simulink model "ME416_Autonomy_Model"  (R2025b)
settings: Solver=FixedStepAuto  StartTime=0.0  StopTime=20  RelTol=1e-3  EnableMultiTasking=on
PreLoadFcn:
  | driveparam
values from neighbouring files (symbols this model uses):
  alpha_w = 0.7    [driveparam.m]
  beta = Ts / (Ts + tau)    (= 0.166666666667)    [driveparam.m]
  bm = 2e-4    (= 0.0002)    [driveparam.m]
  enable_cmd = 1    [driveparam.m]
  estop_cmd = 0    [driveparam.m]
  Jm = 2e-5    (= 2e-05)    [driveparam.m]
  K_lqr_w = dlqr(Ad_w, Bd_w, Qw, Rw)    [driveparam.m]
  Ke = 0.03    [driveparam.m]
  Kt = 0.03    [driveparam.m]
  L = 0.15    [driveparam.m]
  Lm = 1    [driveparam.m]
  N = 4400    [driveparam.m]
  Nbar_lqr_w = (1 - Ad_w)/Bd_w + K_lqr_w    [driveparam.m]
  r = 0.03    [driveparam.m]
  Rm = 8    [driveparam.m]
  Ts = 0.01    [driveparam.m]
  v_ref_cmd = 0    [driveparam.m]
  Vbatt = 12    [driveparam.m]
  w_ref_cmd = 0.1    [driveparam.m]
undefined symbols (not defined in the file or in its folder): DiscIntNeverNeededParam
libraries: raspberrypiBasiclib x10, raspberrypiCommlib x5, simulink x4, slpidlib x2
settings Model: ExtModeTrigDuration=2  Creator=madak  LastModifiedBy=madak
settings SolverCC: PositivePriorityOrder=on  AutoInsertRateTranBlk=on
settings OptimizationCC: DefaultParameterBehavior=Inlined  EnhancedBackFolding=on  PassReuseOutputArgsAs=Individual arguments  ZeroExternalMemoryAtStartup=off  ZeroInternalMemoryAtStartup=off  MaxStackSize=200000  OptimizeBlockOrder=speed  DifferentSizesBufferReuse=on  OptimizationCustomize=off  EfficientTunableParamExpr=on
settings DebuggingCC: ParameterPrecisionLossMsg=none  ParameterTunabilityLossMsg=error
settings HardwareCC: ProdBitPerLong=64.0  ProdLargestAtomicInteger=LongLong  ProdLargestAtomicFloat=Double  ProdLongLongMode=on  ProdHWDeviceType=ARM Compatible->ARM Cortex-A (64-bit)
settings RTWCC: SystemTargetFile=ert.tlc  HardwareBoard=Raspberry Pi (64bit)  TLCOptions="-aInlineSetEventsForThisBaseRateFcn=TLC_FALSE -aSuppressMultiTaskScheduler=TLC_FALSE  -aRateBasedStepFcn=0"  TemplateMakefile=ert_default_tmf  Toolchain=GNU GCC Embedded Linux  BuildConfiguration=Faster Runs  GPUComputeCapability=3.5  Description=Embedded Coder
settings CodeAppCC: ForceParamTrailComments=on  IgnoreCustomStorageClasses=off  OperatorAnnotations=on  SimulinkDataObjDesc=on  SFDataObjDesc=on  InsertBlockDesc=on
settings ERTTargetCC: ExtModeTransport=2.0  ExtModeStaticAlloc=on  ExtModeMexFile=ext_xcp  ExtModeIntrfLevel=Level2 - Open  RootIOFormat=Structure reference  DynamicArrayContainerType=coder::array  TargetLangStandard=C99 (ISO)  SupportContinuousTime=on  SupportVariableSizeSignals=on

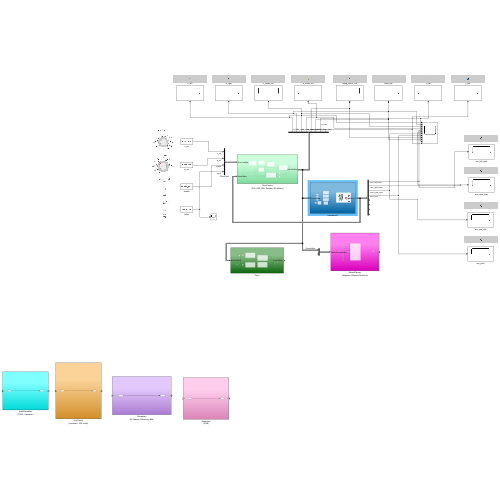
[thumbnail: Simulink's stored preview of the top-level diagram]
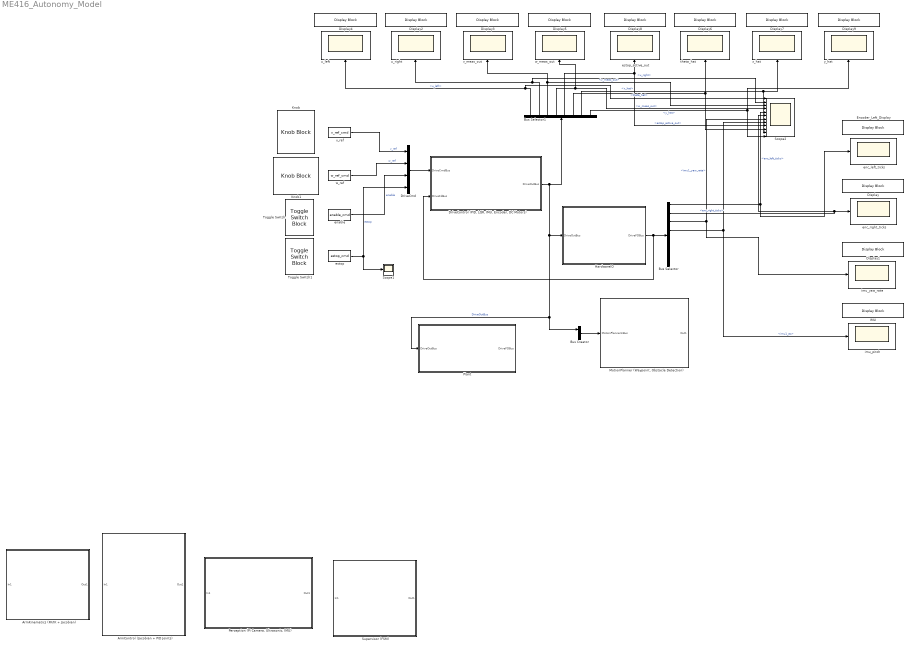
== system ME416_Autonomy_Model ==
  ArmControl (Jacobian + PID Joints) : Subsystem
  ArmKinematics (FK/IK + Jacobian) : Subsystem
  Bus Creator : BusCreator  Inputs=2
  Bus Selector : BusSelector  OutputSignals=enc_left_ticks,enc_right_ticks,imu1_yaw_rate,imu1_az,imu1_ay,imu1_ax,imu1_roll,imu1_pitch
  Bus Selector1 : BusSelector  OutputSignals=u_left,u_right,v_meas_out,w_meas_out,estop_active_out,theta_hat,x_hat,y_hat
  Display{,1..9} (10 alike) : DisplayBlock  LabelPosition=Hide  Transparency=1  GridColor=[0.502, 0.502, 0.502]
  DriveCmd : BusCreator  Inputs=4
  "DriveControl (PID, LQR, IMU, Encoder, DC Motors)" : Subsystem
  Encoder_Left_Display : DisplayBlock  LabelPosition=Hide  Transparency=1  GridColor=[0.502, 0.502, 0.502]
  HardwareIO : Subsystem
  IMU : DisplayBlock  LabelPosition=Hide  Transparency=1  GridColor=[0.502, 0.502, 0.502]
  Knob : KnobBlock  ScaleMin=-0.5  ScaleMax=0.5  TickInterval=0.1
  Knob1 : KnobBlock  ScaleMin=-1  ScaleMax=1
  "MotionPlanner (Waypoint, Obstacle Detection)" : Subsystem
  "Perception (Pi Camera, Ultrasonic, IMU)" : Subsystem
  Plant : Subsystem
  Scope1 : Scope
      settings: ActiveDisplayYMinimum=-1  ActiveDisplayYMaximum=1  DataLoggingVariableName=ScopeData6
  Scope2 : Scope  NumInputPorts=12
      settings: ActiveDisplayYMinimum=-1.25  ActiveDisplayYMaximum=1.25
  Supervisor (FSM) : Subsystem
  Toggle Switch : ToggleSwitchBlock
  Toggle Switch1 : ToggleSwitchBlock
  enable : Constant  Value=enable_cmd
  enc_left_ticks : Scope
      settings: ActiveDisplayYMinimum=-6650.75  ActiveDisplayYMaximum=55596.75
  enc_right_ticks : Scope
      settings: ActiveDisplayYMinimum=-6176.5  ActiveDisplayYMaximum=50648.5  DataLoggingVariableName=ScopeData2
  estop : Constant  Value=estop_cmd  OutDataTypeStr=boolean
  estop_active_out : Scope
      settings: ActiveDisplayYMinimum=-1.25  ActiveDisplayYMaximum=1.25
  imu_pitch : Scope
      settings: ActiveDisplayYMinimum=-1  ActiveDisplayYMaximum=1  DataLoggingVariableName=ScopeData4
  imu_yaw_rate : Scope
      settings: ActiveDisplayYMinimum=-1  ActiveDisplayYMaximum=1  DataLoggingVariableName=ScopeData3
  theta_hat : Scope
      settings: ActiveDisplayYMinimum=-1.25  ActiveDisplayYMaximum=1.25  DataLoggingVariableName=ScopeData2
  u_left : Scope
      settings: ActiveDisplayYMinimum=-1.25  ActiveDisplayYMaximum=1.25
  u_right : Scope
      settings: ActiveDisplayYMinimum=-1.25  ActiveDisplayYMaximum=1.25  DataLoggingVariableName=ScopeData2
  v_meas_out : Scope
      settings: ActiveDisplayYMinimum=-0.06499  ActiveDisplayYMaximum=0.58495  DataLoggingVariableName=ScopeData3
  v_ref : Constant  Value=v_ref_cmd
  w_meas_out : Scope
      settings: ActiveDisplayYMinimum=-29.4564  ActiveDisplayYMaximum=29.55132  DataLoggingVariableName=ScopeData4
  w_ref : Constant  Value=w_ref_cmd
  x_hat : Scope
      settings: ActiveDisplayYMinimum=-6600.125  ActiveDisplayYMaximum=55141.125  DataLoggingVariableName=ScopeData3
  y_hat : Scope
      settings: ActiveDisplayYMinimum=-29.4564  ActiveDisplayYMaximum=29.55132  DataLoggingVariableName=ScopeData4
  wires:
  DriveCmd/1 -> "DriveControl (PID, LQR, IMU, Encoder, DC Motors)"/1(DriveCmdBus)
  "DriveControl (PID, LQR, IMU, Encoder, DC Motors)"/1(DriveOutBus) -> Bus Creator/1, Plant/1(DriveOutBus), HardwareIO/1(DriveOutBus), Bus Selector1/1  "DriveOutBus"
  v_ref/1 -> DriveCmd/1  "v_ref"
  w_ref/1 -> DriveCmd/2  "w_ref"
  enable/1 -> DriveCmd/3  "enable"
  estop/1 -> DriveCmd/4, Scope1/1  "estop"
  Bus Selector/1 -> enc_left_ticks/1, Scope2/5  "<enc_left_ticks>"
  Bus Selector/2 -> Scope2/6, enc_right_ticks/1  "<enc_right_ticks>"
  Bus Selector1/1 -> Scope2/1, u_left/1  "<u_left>"
  Bus Selector1/2 -> Scope2/2, u_right/1  "<u_right>"
  Bus Selector1/3 -> Scope2/3, v_meas_out/1  "<v_meas_out>"
  Bus Selector1/4 -> Scope2/4, w_meas_out/1  "<w_meas_out>"
  Bus Creator/1 -> "MotionPlanner (Waypoint, Obstacle Detection)"/1(MotionPlannerInBus)
  Bus Selector1/5 -> Scope2/9, estop_active_out/1  "<estop_active_out>"
  Bus Selector1/6 -> Scope2/10, theta_hat/1  "<theta_hat>"
  Bus Selector1/7 -> Scope2/11, x_hat/1  "<x_hat>"
  Bus Selector1/8 -> y_hat/1, Scope2/12  "<y_hat>"
  HardwareIO/1("DriveFDBus ") -> "DriveControl (PID, LQR, IMU, Encoder, DC Motors)"/2(DriveFdBus), Bus Selector/1
  Bus Selector/3 -> imu_yaw_rate/1, Scope2/7  "<imu1_yaw_rate>"
  Bus Selector/4 -> imu_pitch/1, Scope2/8  "<imu1_az>"

== system ME416_Autonomy_Model/ArmControl (Jacobian + PID Joints) ==
  In1 : Inport
  Out1 : Outport
  wires:
  In1/1 -> Out1/1

== system ME416_Autonomy_Model/ArmKinematics (FK//IK + Jacobian) ==
  In1 : Inport
  Out1 : Outport
  wires:
  In1/1 -> Out1/1

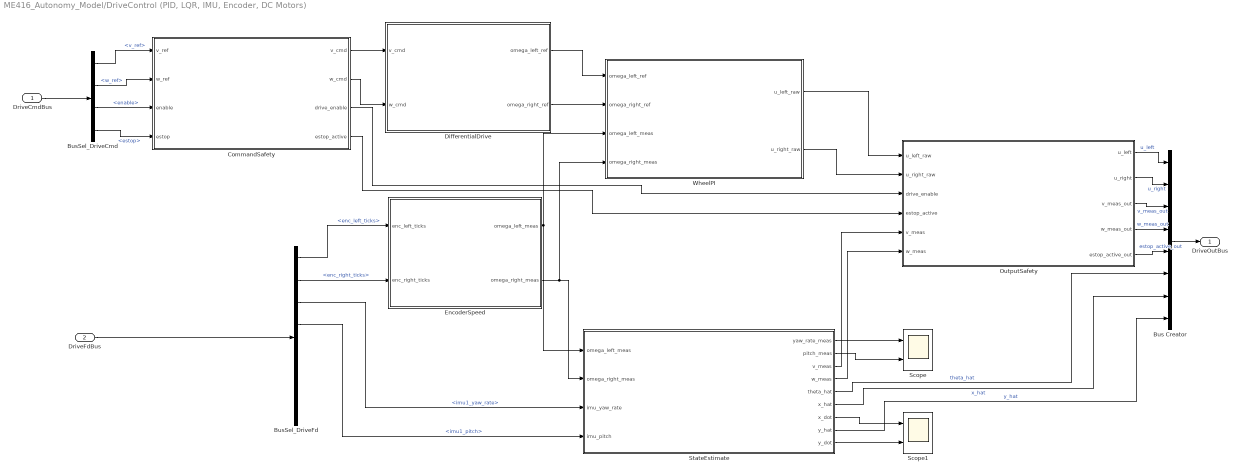
== system ME416_Autonomy_Model/DriveControl (PID, LQR, IMU, Encoder, DC Motors) ==
  DriveCmdBus : Inport
  DriveFdBus : Inport  Port=2
  Bus Creator : BusCreator  Inputs=8
  BusSel_DriveCmd : BusSelector  OutputSignals=v_ref,w_ref,enable,estop
  BusSel_DriveFd : BusSelector  OutputSignals=enc_left_ticks,enc_right_ticks,imu1_yaw_rate,imu1_pitch,imu1_roll,imu1_ax,imu1_ay,imu1_az
  CommandSafety : Subsystem
  DifferentialDrive : Subsystem
  EncoderSpeed : Subsystem
  OutputSafety : Subsystem
  Scope : Scope  NumInputPorts=2
      settings: ActiveDisplayYMinimum=-1  ActiveDisplayYMaximum=1
  Scope1 : Scope  NumInputPorts=2
      settings: ActiveDisplayYMinimum=-1  ActiveDisplayYMaximum=1
  StateEstimate : Subsystem
  WheelPI : Subsystem
  DriveOutBus : Outport
  wires:
  DriveCmdBus/1 -> BusSel_DriveCmd/1
  StateEstimate/4(w_meas) -> OutputSafety/6(w_meas)
  DriveFdBus/1 -> BusSel_DriveFd/1
  StateEstimate/6(x_hat) -> Bus Creator/7  "x_hat"
  BusSel_DriveCmd/1 -> CommandSafety/1(v_ref)  "<v_ref>"
  CommandSafety/2(w_cmd) -> DifferentialDrive/2(w_cmd)
  BusSel_DriveCmd/2 -> CommandSafety/2(w_ref)  "<w_ref>"
  BusSel_DriveCmd/4 -> CommandSafety/4(estop)  "<estop>"
  BusSel_DriveCmd/3 -> CommandSafety/3(enable)  "<enable>"
  CommandSafety/1(v_cmd) -> DifferentialDrive/1(v_cmd)
  CommandSafety/3(drive_enable) -> OutputSafety/3(drive_enable)
  CommandSafety/4(estop_active) -> OutputSafety/4(estop_active)
  StateEstimate/3(v_meas) -> OutputSafety/5(v_meas)
  BusSel_DriveFd/1 -> EncoderSpeed/1(enc_left_ticks)  "<enc_left_ticks>"
  BusSel_DriveFd/2 -> EncoderSpeed/2(enc_right_ticks)  "<enc_right_ticks>"
  BusSel_DriveFd/3 -> StateEstimate/3(imu_yaw_rate)  "<imu1_yaw_rate>"
  BusSel_DriveFd/4 -> StateEstimate/4(imu_pitch)  "<imu1_pitch>"
  DifferentialDrive/1(omega_left_ref) -> WheelPI/1(omega_left_ref)
  DifferentialDrive/2(omega_right_ref) -> WheelPI/2(omega_right_ref)
  EncoderSpeed/1(omega_left_meas) -> StateEstimate/1(omega_left_meas), WheelPI/3(omega_left_meas)
  EncoderSpeed/2(omega_right_meas) -> WheelPI/4(omega_right_meas), StateEstimate/2(omega_right_meas)
  WheelPI/1(u_left_raw) -> OutputSafety/1(u_left_raw)
  WheelPI/2(u_right_raw) -> OutputSafety/2(u_right_raw)
  Bus Creator/1 -> DriveOutBus/1
  StateEstimate/9(y_dot) -> Scope1/2
  StateEstimate/1(yaw_rate_meas) -> Scope/1
  StateEstimate/2(pitch_meas) -> Scope/2
  StateEstimate/5(theta_hat) -> Bus Creator/6  "theta_hat"
  StateEstimate/7(x_dot) -> Scope1/1
  StateEstimate/8(y_hat) -> Bus Creator/8  "y_hat"
  OutputSafety/1(u_left) -> Bus Creator/1  "u_left"
  OutputSafety/2(u_right) -> Bus Creator/2  "u_right"
  OutputSafety/3(v_meas_out) -> Bus Creator/3  "v_meas_out"
  OutputSafety/4(w_meas_out) -> Bus Creator/4  "w_meas_out"
  OutputSafety/5(estop_active_out) -> Bus Creator/5  "estop_active_out"

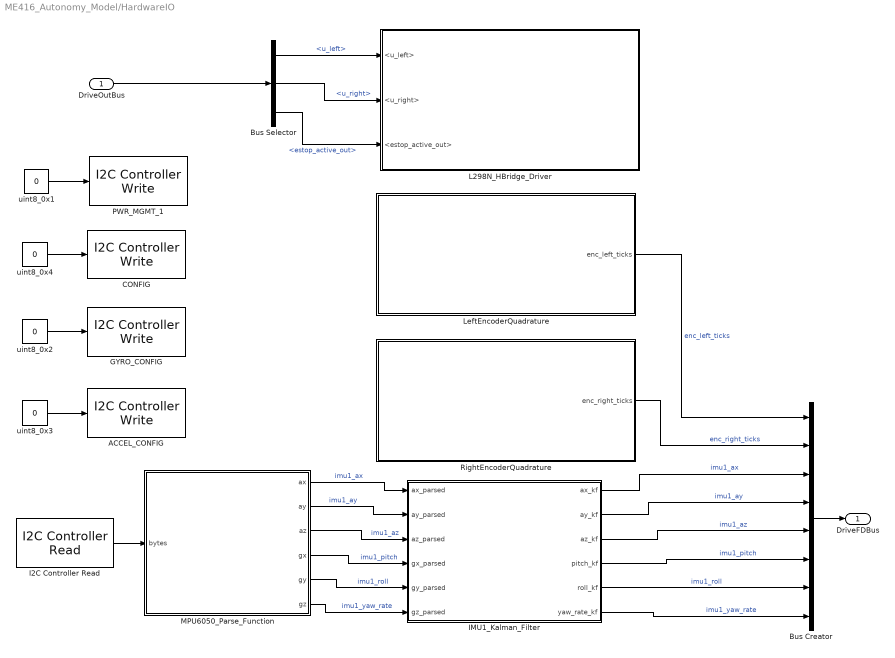
== system ME416_Autonomy_Model/HardwareIO ==
  DriveOutBus : Inport
  ACCEL_CONFIG : raspberrypiCommlib/I2C Controller Write  BoardProperty=Pi 4 Model B  I2CModule=1  Mode=Master  SlaveAddress=0x68  SlaveByteOrder=BigEndian  Direction=Transmitter  RegisterAddressMode=on  RegisterAddress=0x1C  SlaveDataType=uint8  DataLength=1  NoAck=off  RepeatedStart=off  OutputStatus=off
  Bus Creator : BusCreator  Inputs=8
  Bus Selector : BusSelector  OutputSignals=u_left,u_right,estop_active_out
  CONFIG : raspberrypiCommlib/I2C Controller Write  BoardProperty=Pi 4 Model B  I2CModule=1  Mode=Master  SlaveAddress=0x68  SlaveByteOrder=BigEndian  Direction=Transmitter  RegisterAddressMode=on  RegisterAddress=0x1A  SlaveDataType=uint8  DataLength=1  NoAck=off  RepeatedStart=off  OutputStatus=off
  GYRO_CONFIG : raspberrypiCommlib/I2C Controller Write  BoardProperty=Pi 4 Model B  I2CModule=1  Mode=Master  SlaveAddress=0x68  SlaveByteOrder=BigEndian  Direction=Transmitter  RegisterAddressMode=on  RegisterAddress=0x1A  SlaveDataType=uint8  DataLength=1  NoAck=off  RepeatedStart=off  OutputStatus=off
  I2C Controller Read : raspberrypiCommlib/I2C Controller Read  BoardProperty=Pi 4 Model B  I2CModule=1  Mode=Master  SlaveAddress=0x68  SlaveByteOrder=BigEndian  Direction=Receiver  RegisterAddressMode=on  RegisterAddress=0x6B  SlaveDataType=uint8  DataLength=14  NoAck=off  RepeatedStart=off  OutputStatus=off  SampleTime=0.01
  IMU1_Kalman_Filter : MATLAB Function  TreatAsAtomicUnit=on
  L298N_HBridge_Driver : Subsystem
  LeftEncoderQuadrature : Subsystem
  MPU6050_Parse_Function : MATLAB Function  TreatAsAtomicUnit=on
  PWR_MGMT_1 : raspberrypiCommlib/I2C Controller Write  BoardProperty=Pi 4 Model B  I2CModule=1  Mode=Master  SlaveAddress=0x68  SlaveByteOrder=BigEndian  Direction=Transmitter  RegisterAddressMode=on  RegisterAddress=0x6B  SlaveDataType=uint8  DataLength=1  NoAck=off  RepeatedStart=off  OutputStatus=off
  RightEncoderQuadrature : Subsystem
  uint8_0x{1..4} (4 alike) : Constant  Value=0  OutDataTypeStr=uint8
  "DriveFDBus " : Outport
  wires:
  uint8_0x1/1 -> PWR_MGMT_1/1
  DriveOutBus/1 -> Bus Selector/1
  MPU6050_Parse_Function/2(ay) -> IMU1_Kalman_Filter/2(ay_parsed)  "imu1_ay"
  Bus Selector/3 -> L298N_HBridge_Driver/3(<estop_active_out>)  "<estop_active_out>"
  Bus Selector/2 -> L298N_HBridge_Driver/2(<u_right>)  "<u_right>"
  MPU6050_Parse_Function/4(gx) -> IMU1_Kalman_Filter/4(gx_parsed)  "imu1_pitch"
  Bus Selector/1 -> L298N_HBridge_Driver/1(<u_left>)  "<u_left>"
  I2C Controller Read/1 -> MPU6050_Parse_Function/1(bytes)
  MPU6050_Parse_Function/1(ax) -> IMU1_Kalman_Filter/1(ax_parsed)  "imu1_ax"
  MPU6050_Parse_Function/3(az) -> IMU1_Kalman_Filter/3(az_parsed)  "imu1_az"
  MPU6050_Parse_Function/5(gy) -> IMU1_Kalman_Filter/5(gy_parsed)  "imu1_roll"
  MPU6050_Parse_Function/6(gz) -> IMU1_Kalman_Filter/6(gz_parsed)  "imu1_yaw_rate"
  LeftEncoderQuadrature/1(enc_left_ticks) -> Bus Creator/1  "enc_left_ticks"
  RightEncoderQuadrature/1(enc_right_ticks) -> Bus Creator/2  "enc_right_ticks"
  IMU1_Kalman_Filter/1(ax_kf) -> Bus Creator/3  "imu1_ax"
  IMU1_Kalman_Filter/2(ay_kf) -> Bus Creator/4  "imu1_ay"
  IMU1_Kalman_Filter/3(az_kf) -> Bus Creator/5  "imu1_az"
  IMU1_Kalman_Filter/4(pitch_kf) -> Bus Creator/6  "imu1_pitch"
  IMU1_Kalman_Filter/5(roll_kf) -> Bus Creator/7  "imu1_roll"
  IMU1_Kalman_Filter/6(yaw_rate_kf) -> Bus Creator/8  "imu1_yaw_rate"
  Bus Creator/1 -> "DriveFDBus "/1
  uint8_0x2/1 -> GYRO_CONFIG/1
  uint8_0x3/1 -> ACCEL_CONFIG/1
  uint8_0x4/1 -> CONFIG/1

== system ME416_Autonomy_Model/MotionPlanner (Waypoint, Obstacle Detection) ==
  MotionPlannerInBus : Inport
  Bus Selector : BusSelector  OutputSignals=DriveOutBus.u_left,DriveOutBus.u_right,DriveOutBus.v_meas_out,DriveOutBus.w_meas_out,DriveOutBus.estop_active_out,DriveOutBus.theta_hat,DriveOutBus.x_hat,DriveOutBus.y_hat
  Subsystem : Subsystem
  Out1 : Outport
  wires:
  MotionPlannerInBus/1 -> Bus Selector/1
  Bus Selector/1 -> Subsystem/1(u_left)  "<u_left>"
  Bus Selector/3 -> Subsystem/3(v_meas_out)  "<v_meas_out>"
  Bus Selector/2 -> Subsystem/2(u_right)  "<u_right>"
  Bus Selector/7 -> Subsystem/7(x_hat)  "<x_hat>"
  Bus Selector/6 -> Subsystem/6(theta_hat)  "<theta_hat>"
  Bus Selector/5 -> Subsystem/5(estop_active_out)  "<estop_active_out>"
  Bus Selector/8 -> Subsystem/8(y_hat)  "<y_hat>"
  Bus Selector/4 -> Subsystem/4(w_meas_out)  "<w_meas_out>"

== system ME416_Autonomy_Model/Perception (Pi Camera, Ultrasonic, IMU) ==
  In1 : Inport
  Out1 : Outport
  wires:
  In1/1 -> Out1/1

== system ME416_Autonomy_Model/Plant ==
  DriveOutBus : Inport
  Bus Creator : BusCreator  Inputs=4
  Bus Selector : BusSelector  OutputSignals=u_left,u_right
  DifferentialDriveModel : Subsystem
  EncoderModel : Subsystem
  MotorDynamics_Left : Subsystem
  MotorDynamics_Right : Subsystem
  V_left_batt : Product
  V_right_batt : Product
  Vbatt : Constant  Value=Vbatt
  "DriveFDBus " : Outport
  wires:
  MotorDynamics_Left/2("omega_left_true ") -> EncoderModel/1(omega_left_true), DifferentialDriveModel/1(omega_true_left)
  DifferentialDriveModel/2(imu_pitch) -> Bus Creator/4  "imu_pitch"
  Vbatt/1 -> V_right_batt/1, V_left_batt/2
  Bus Selector/1 -> V_left_batt/1  "<u_left>"
  Bus Selector/2 -> V_right_batt/2  "<u_right>"
  V_left_batt/1 -> MotorDynamics_Left/1(V_left)
  V_right_batt/1 -> MotorDynamics_Right/1(V_right)
  MotorDynamics_Right/2("omega_right_true ") -> DifferentialDriveModel/2(omega_true_right), EncoderModel/2(omega_right_true)
  EncoderModel/1(enc_left_ticks) -> Bus Creator/1  "enc_left_ticks"
  EncoderModel/2(enc_right_ticks) -> Bus Creator/2  "enc_right_ticks"
  DifferentialDriveModel/1(imu_yaw_rate) -> Bus Creator/3  "imu_yaw_rate"
  Bus Creator/1 -> "DriveFDBus "/1
  DriveOutBus/1 -> Bus Selector/1

== system ME416_Autonomy_Model/Supervisor (FSM) ==
  In1 : Inport
  Out1 : Outport
  wires:
  In1/1 -> Out1/1

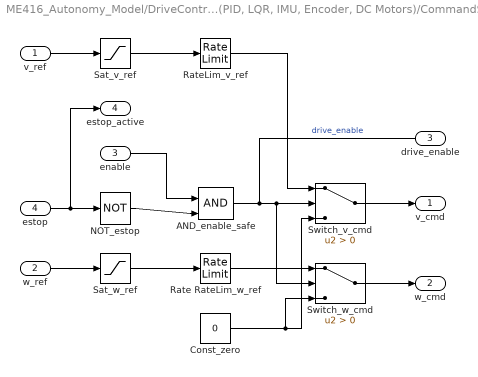
== system ME416_Autonomy_Model/DriveControl (PID, LQR, IMU, Encoder, DC Motors)/CommandSafety ==
  v_ref : Inport
  w_ref : Inport  Port=2
  enable : Inport  Port=3
  estop : Inport  Port=4
  AND_enable_safe : Logic  IconShape=distinctive  AllPortsSameDT=off  OutDataTypeStr=boolean
  Const_zero : Constant  Value=0
  NOT_estop : Logic  Operator=NOT  IconShape=distinctive  AllPortsSameDT=off  OutDataTypeStr=boolean
  Rate RateLim_w_ref : RateLimiter  SampleTimeMode=inherited
  RateLim_v_ref : RateLimiter  SampleTimeMode=inherited
  Sat_v_ref : Saturate  UpperLimit=0.6  LowerLimit=-0.6
  Sat_w_ref : Saturate  UpperLimit=1.5  LowerLimit=-1.5
  Switch_v_cmd : Switch  Criteria=u2 > Threshold  SaturateOnIntegerOverflow=off  InputSameDT=off
  Switch_w_cmd : Switch  Criteria=u2 > Threshold  SaturateOnIntegerOverflow=off  InputSameDT=off
  v_cmd : Outport
  w_cmd : Outport  Port=2
  drive_enable : Outport  Port=3
  estop_active : Outport  Port=4
  wires:
  v_ref/1 -> Sat_v_ref/1
  estop/1 -> NOT_estop/1, estop_active/1
  Sat_w_ref/1 -> Rate RateLim_w_ref/1
  w_ref/1 -> Sat_w_ref/1
  NOT_estop/1 -> AND_enable_safe/2
  Sat_v_ref/1 -> RateLim_v_ref/1
  enable/1 -> AND_enable_safe/1
  RateLim_v_ref/1 -> Switch_v_cmd/1
  AND_enable_safe/1 -> Switch_w_cmd/2, Switch_v_cmd/2, drive_enable/1  "drive_enable"
  Rate RateLim_w_ref/1 -> Switch_w_cmd/1
  Const_zero/1 -> Switch_v_cmd/3, Switch_w_cmd/3
  Switch_v_cmd/1 -> v_cmd/1
  Switch_w_cmd/1 -> w_cmd/1

== system ME416_Autonomy_Model/DriveControl (PID, LQR, IMU, Encoder, DC Motors)/DifferentialDrive ==
  v_cmd : Inport
  w_cmd : Inport  Port=2
  Gain_inv_r_left : Gain  Gain=1/r
  Product : Product
  Sum_v_left : Sum  Inputs=+-
  Sum_v_right : Sum
  gain_inv_r_right : Gain  Gain=1/r
  w_term : Constant  Value=L/2
  omega_left_ref : Outport
  omega_right_ref : Outport  Port=2
  wires:
  w_term/1 -> Product/1
  gain_inv_r_right/1 -> omega_right_ref/1
  w_cmd/1 -> Product/2
  v_cmd/1 -> Sum_v_right/1, Sum_v_left/1
  Sum_v_right/1 -> gain_inv_r_right/1  "v_right"
  Product/1 -> Sum_v_left/2, Sum_v_right/2
  Gain_inv_r_left/1 -> omega_left_ref/1
  Sum_v_left/1 -> Gain_inv_r_left/1  "v_left"

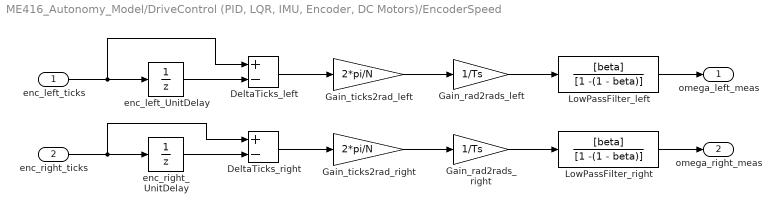
== system ME416_Autonomy_Model/DriveControl (PID, LQR, IMU, Encoder, DC Motors)/EncoderSpeed ==
  enc_left_ticks : Inport
  enc_right_ticks : Inport  Port=2
  DeltaTicks_left : Sum  Inputs=+-
  DeltaTicks_right : Sum  Inputs=+-
  Gain_rad2rads_left : Gain  Gain=1/Ts
  Gain_rad2rads_right : Gain  Gain=1/Ts
  Gain_ticks2rad_left : Gain  Gain=2*pi/N
  Gain_ticks2rad_right : Gain  Gain=2*pi/N
  LowPassFilter_left : DiscreteTransferFcn  Numerator=[beta]  Denominator=[1 -(1 - beta)]  SampleTime=Ts
  LowPassFilter_right : DiscreteTransferFcn  Numerator=[beta]  Denominator=[1 -(1 - beta)]  SampleTime=Ts
  enc_left_UnitDelay : UnitDelay  SampleTime=-1  HasFrameUpgradeWarning=on
  enc_right_UnitDelay : UnitDelay  SampleTime=-1  HasFrameUpgradeWarning=on
  omega_left_meas : Outport
  omega_right_meas : Outport  Port=2
  wires:
  enc_left_ticks/1 -> DeltaTicks_left/1, enc_left_UnitDelay/1
  Gain_ticks2rad_right/1 -> Gain_rad2rads_right/1
  enc_right_ticks/1 -> DeltaTicks_right/1, enc_right_UnitDelay/1
  enc_right_UnitDelay/1 -> DeltaTicks_right/2
  enc_left_UnitDelay/1 -> DeltaTicks_left/2
  DeltaTicks_left/1 -> Gain_ticks2rad_left/1
  DeltaTicks_right/1 -> Gain_ticks2rad_right/1
  Gain_ticks2rad_left/1 -> Gain_rad2rads_left/1
  Gain_rad2rads_left/1 -> LowPassFilter_left/1
  Gain_rad2rads_right/1 -> LowPassFilter_right/1
  LowPassFilter_left/1 -> omega_left_meas/1
  LowPassFilter_right/1 -> omega_right_meas/1

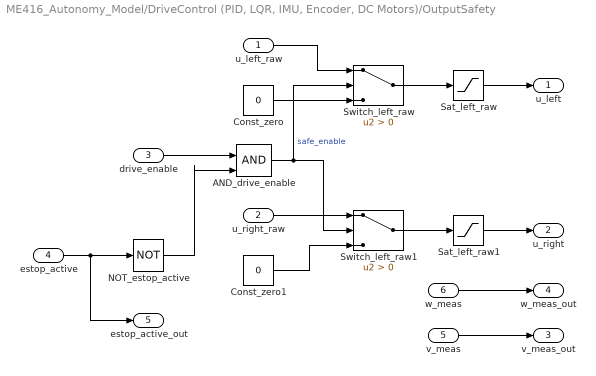
== system ME416_Autonomy_Model/DriveControl (PID, LQR, IMU, Encoder, DC Motors)/OutputSafety ==
  u_left_raw : Inport
  u_right_raw : Inport  Port=2
  drive_enable : Inport  Port=3
  estop_active : Inport  Port=4
  v_meas : Inport  Port=5
  w_meas : Inport  Port=6
  AND_drive_enable : Logic  IconShape=distinctive  AllPortsSameDT=off  OutDataTypeStr=boolean
  Const_zero : Constant  Value=0
  Const_zero1 : Constant  Value=0
  NOT_estop_active : Logic  Operator=NOT  IconShape=distinctive  AllPortsSameDT=off  OutDataTypeStr=boolean
  Sat_left_raw : Saturate  UpperLimit=1  LowerLimit=-1
  Sat_left_raw1 : Saturate  UpperLimit=1  LowerLimit=-1
  Switch_left_raw : Switch  Criteria=u2 > Threshold  SaturateOnIntegerOverflow=off  InputSameDT=off
  Switch_left_raw1 : Switch  Criteria=u2 > Threshold  SaturateOnIntegerOverflow=off  InputSameDT=off
  u_left : Outport
  u_right : Outport  Port=2
  v_meas_out : Outport  Port=3
  w_meas_out : Outport  Port=4
  estop_active_out : Outport  Port=5
  wires:
  u_left_raw/1 -> Switch_left_raw/1
  w_meas/1 -> w_meas_out/1
  v_meas/1 -> v_meas_out/1
  AND_drive_enable/1 -> Switch_left_raw1/2, Switch_left_raw/2  "safe_enable"
  estop_active/1 -> estop_active_out/1, NOT_estop_active/1
  drive_enable/1 -> AND_drive_enable/1
  NOT_estop_active/1 -> AND_drive_enable/2
  Const_zero/1 -> Switch_left_raw/3
  u_right_raw/1 -> Switch_left_raw1/1
  Const_zero1/1 -> Switch_left_raw1/3
  Switch_left_raw/1 -> Sat_left_raw/1
  Switch_left_raw1/1 -> Sat_left_raw1/1
  Sat_left_raw/1 -> u_left/1
  Sat_left_raw1/1 -> u_right/1

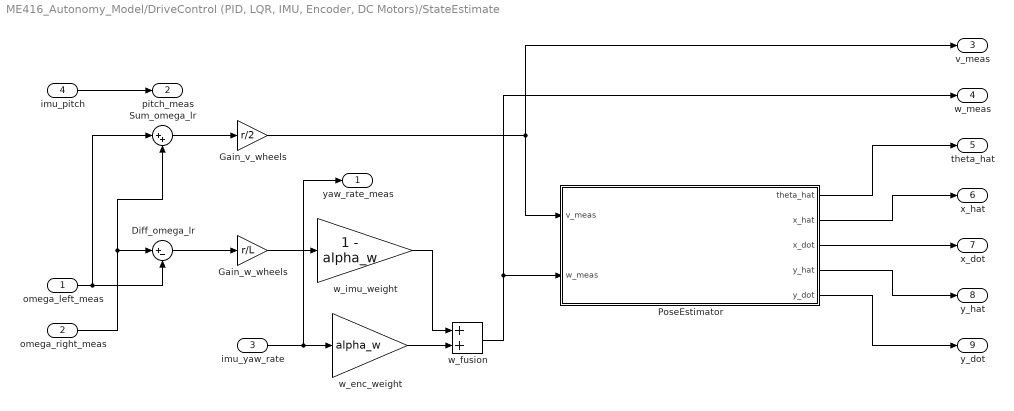
== system ME416_Autonomy_Model/DriveControl (PID, LQR, IMU, Encoder, DC Motors)/StateEstimate ==
  omega_left_meas : Inport
  omega_right_meas : Inport  Port=2
  imu_yaw_rate : Inport  Port=3
  imu_pitch : Inport  Port=4
  Diff_omega_lr : Sum  Inputs=|+-
  Gain_v_wheels : Gain  Gain=r/2
  Gain_w_wheels : Gain  Gain=r/L
  PoseEstimator : Subsystem
  Sum_omega_lr : Sum  Inputs=|++
  w_enc_weight : Gain  Gain=alpha_w
  w_fusion : Sum
  w_imu_weight : Gain  Gain=1 - alpha_w
  yaw_rate_meas : Outport
  pitch_meas : Outport  Port=2
  v_meas : Outport  Port=3
  w_meas : Outport  Port=4
  theta_hat : Outport  Port=5
  x_hat : Outport  Port=6
  x_dot : Outport  Port=7
  y_hat : Outport  Port=8
  y_dot : Outport  Port=9
  wires:
  omega_right_meas/1 -> Diff_omega_lr/1, Sum_omega_lr/2
  imu_pitch/1 -> pitch_meas/1
  imu_yaw_rate/1 -> yaw_rate_meas/1, w_enc_weight/1
  Gain_w_wheels/1 -> w_imu_weight/1
  omega_left_meas/1 -> Sum_omega_lr/1, Diff_omega_lr/2
  Sum_omega_lr/1 -> Gain_v_wheels/1
  Diff_omega_lr/1 -> Gain_w_wheels/1
  w_imu_weight/1 -> w_fusion/1
  w_enc_weight/1 -> w_fusion/2
  w_fusion/1 -> w_meas/1, PoseEstimator/2(w_meas)
  PoseEstimator/1(theta_hat) -> theta_hat/1
  PoseEstimator/2(x_hat) -> x_hat/1
  PoseEstimator/3(x_dot) -> x_dot/1
  PoseEstimator/4(y_hat) -> y_hat/1
  PoseEstimator/5(y_dot) -> y_dot/1
  Gain_v_wheels/1 -> PoseEstimator/1(v_meas), v_meas/1

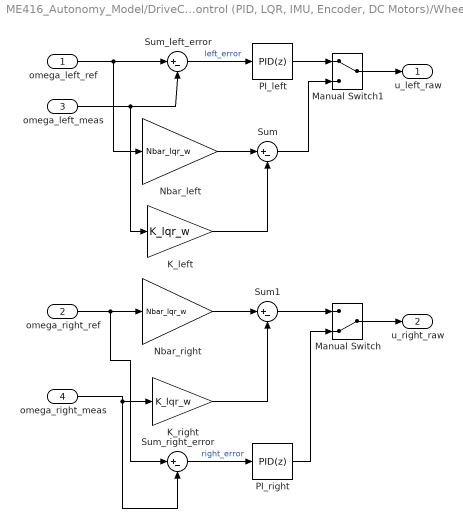
== system ME416_Autonomy_Model/DriveControl (PID, LQR, IMU, Encoder, DC Motors)/WheelPI ==
  omega_left_ref : Inport
  omega_right_ref : Inport  Port=2
  omega_left_meas : Inport  Port=3
  omega_right_meas : Inport  Port=4
  K_left : Gain  Gain=K_lqr_w
  K_right : Gain  Gain=K_lqr_w
  Manual Switch : ManualSwitch  CurrentSetting=0
  Manual Switch1 : ManualSwitch
  Nbar_left : Gain  Gain=Nbar_lqr_w
  Nbar_right : Gain  Gain=Nbar_lqr_w
  PI_left : slpidlib/PID Controller  Controller=PID  Form=Parallel  TimeDomain=Discrete-time  UseExternalTs=off  SampleTime=0.01  IntegratorMethod=Forward Euler  FilterMethod=Forward Euler  ControllerParametersSource=internal  P=0.02711  I=0.00415  UseKiTs=off  D=0  UseExternalDerivativeSource=off  N=100  UseFilter=on  TunerSelectOption=Frequency Response Based  InitialConditionSource=internal  InitialConditionForIntegrator=0  InitialConditionForFilter=0  DifferentiatorICPrevScaledInput=0  ExternalReset=none  TrackingMode=off  Kt=1  LimitOutput=off  SatLimitsSource=internal  UpperSaturationLimit=inf  LowerSaturationLimit=-inf  LinearizeAsGain=off  AntiWindupMode=none  Kb=1  LimitIntegrator=off  UpperIntegratorSaturationLimit=inf  LowerIntegratorSaturationLimit=-inf  POutMin=[]  POutMax=[]  IOutMin=[]  IOutMax=[]  DOutMin=[]  DOutMax=[]  NOutMin=[]  NOutMax=[]  SumOutMin=[]  SumOutMax=[]  SaturationOutMin=[]  SaturationOutMax=[]  PParamMin=[]  PParamMax=[]  IParamMin=[]  IParamMax=[]  DParamMin=[]  DParamMax=[]  NParamMin=[]  NParamMax=[]  KbParamMin=[]  KbParamMax=[]  KtParamMin=[]  KtParamMax=[]  KbOutMin=[]  KbOutMax=[]  KtOutMin=[]  KtOutMax=[]  IntegratorOutMin=[]  IntegratorOutMax=[]  FilterOutMin=[]  FilterOutMax=[]  SumI1OutMin=[]  SumI1OutMax=[]  SumI2OutMin=[]  SumI2OutMax=[]  SumI3OutMin=[]  SumI3OutMax=[]  SumI4OutMin=[]  SumI4OutMax=[]  SumDOutMin=[]  SumDOutMax=[]  DifferentiatorOutMin=[]  DifferentiatorOutMax=[]  FilterDiffOutCoefMin=[]  FilterDiffOutCoefMax=[]  ReciprocalOutMin=[]  ReciprocalOutMax=[]  SumDenOutMin=[]  SumDenOutMax=[]  SumNumOutMin=[]  SumNumOutMax=[]  DivideOutMin=[]  DivideOutMax=[]  UdiffTsProdOutMin=[]  UdiffTsProdOutMax=[]  NTsProdOutMin=[]  NTsProdOutMax=[]  UintegralTsProdOutMin=[]  UintegralTsProdOutMax=[]  UngainTsProdOutMin=[]  UngainTsProdOutMax=[]  ClampingZeroOutDataTypeStr=Inherit: Inherit via back propagation  ClampingZeroOutMin=[]  ClampingZeroOutMax=[]  FilterDenConstantOutDataTypeStr=Inherit: Inherit via back propagation  FilterDenConstantOutMin=[]  FilterDenConstantOutMax=[]  PCopyOutDataTypeStr=Inherit: Inherit via back propagation  PCopyOutMin=[]  PCopyOutMax=[]  NCopyOutDataTypeStr=Inherit: Inherit via back propagation  NCopyOutMin=[]  NCopyOutMax=[]  IntegratorContinuousStateAttributes=''  IntegratorStateMustResolveToSignalObject=off  IntegratorRTWStateStorageClass=Auto  FilterContinuousStateAttributes=''  FilterStateMustResolveToSignalObject=off  FilterRTWStateStorageClass=Auto  ParallelPVariant=InternalParameters  IdealPVariant=Disabled  IVariant=InternalParameters  DVariant=InternalParameters  IntegratorVariant=Discrete  SatVariant=Disabled  AWVariant=Passthrough  PCopyVariant=Disabled  TRVariant=Disabled  FdbkBlocksVariant=Forward  IdealPFdbkVariant=Disabled  SatFdbkVariant=Disabled  DerivativeFilterVariant=ForwardEulerFilter  NVariant=InternalParameters  NCopyVariant=Disabled  FilterICVariant=InternalICsFilter  IntegratorICVariant=InternalICs  ExternalResetVariant=Disabled  TRSumVariant=Passthrough  SumFdbkVariant=Disabled  SumVariant=Sum_PID  TsampFilterVariant=InternalTs  TsampNgainVariant=Passthrough  TsampIntegralVariant=Disabled_SignalSpec  ExternalSaturationOutDataTypeStr=Inherit: Same as second input  DerivativeSourceVariant=ErrorSignal  PreIntVariant=InternalPreInt
      settings: LibrarySourceBlock=simulink/Discrete/Discrete PID Controller
  PI_right : slpidlib/PID Controller  Controller=PID  Form=Parallel  TimeDomain=Discrete-time  UseExternalTs=off  SampleTime=0.01  IntegratorMethod=Forward Euler  FilterMethod=Forward Euler  ControllerParametersSource=internal  P=0.02711  I=0.00415  UseKiTs=off  D=0  UseExternalDerivativeSource=off  N=100  UseFilter=on  TunerSelectOption=Transfer Function Based (PID Tuner App)  InitialConditionSource=internal  InitialConditionForIntegrator=0  InitialConditionForFilter=0  DifferentiatorICPrevScaledInput=0  ExternalReset=none  TrackingMode=off  Kt=1  LimitOutput=off  SatLimitsSource=internal  UpperSaturationLimit=inf  LowerSaturationLimit=-inf  LinearizeAsGain=off  AntiWindupMode=none  Kb=1  LimitIntegrator=off  UpperIntegratorSaturationLimit=inf  LowerIntegratorSaturationLimit=-inf  POutMin=[]  POutMax=[]  IOutMin=[]  IOutMax=[]  DOutMin=[]  DOutMax=[]  NOutMin=[]  NOutMax=[]  SumOutMin=[]  SumOutMax=[]  SaturationOutMin=[]  SaturationOutMax=[]  PParamMin=[]  PParamMax=[]  IParamMin=[]  IParamMax=[]  DParamMin=[]  DParamMax=[]  NParamMin=[]  NParamMax=[]  KbParamMin=[]  KbParamMax=[]  KtParamMin=[]  KtParamMax=[]  KbOutMin=[]  KbOutMax=[]  KtOutMin=[]  KtOutMax=[]  IntegratorOutMin=[]  IntegratorOutMax=[]  FilterOutMin=[]  FilterOutMax=[]  SumI1OutMin=[]  SumI1OutMax=[]  SumI2OutMin=[]  SumI2OutMax=[]  SumI3OutMin=[]  SumI3OutMax=[]  SumI4OutMin=[]  SumI4OutMax=[]  SumDOutMin=[]  SumDOutMax=[]  DifferentiatorOutMin=[]  DifferentiatorOutMax=[]  FilterDiffOutCoefMin=[]  FilterDiffOutCoefMax=[]  ReciprocalOutMin=[]  ReciprocalOutMax=[]  SumDenOutMin=[]  SumDenOutMax=[]  SumNumOutMin=[]  SumNumOutMax=[]  DivideOutMin=[]  DivideOutMax=[]  UdiffTsProdOutMin=[]  UdiffTsProdOutMax=[]  NTsProdOutMin=[]  NTsProdOutMax=[]  UintegralTsProdOutMin=[]  UintegralTsProdOutMax=[]  UngainTsProdOutMin=[]  UngainTsProdOutMax=[]  ClampingZeroOutDataTypeStr=Inherit: Inherit via back propagation  ClampingZeroOutMin=[]  ClampingZeroOutMax=[]  FilterDenConstantOutDataTypeStr=Inherit: Inherit via back propagation  FilterDenConstantOutMin=[]  FilterDenConstantOutMax=[]  PCopyOutDataTypeStr=Inherit: Inherit via back propagation  PCopyOutMin=[]  PCopyOutMax=[]  NCopyOutDataTypeStr=Inherit: Inherit via back propagation  NCopyOutMin=[]  NCopyOutMax=[]  IntegratorContinuousStateAttributes=''  IntegratorStateMustResolveToSignalObject=off  IntegratorRTWStateStorageClass=Auto  FilterContinuousStateAttributes=''  FilterStateMustResolveToSignalObject=off  FilterRTWStateStorageClass=Auto  ParallelPVariant=InternalParameters  IdealPVariant=Disabled  IVariant=InternalParameters  DVariant=InternalParameters  IntegratorVariant=Discrete  SatVariant=Disabled  AWVariant=Passthrough  PCopyVariant=Disabled  TRVariant=Disabled  FdbkBlocksVariant=Forward  IdealPFdbkVariant=Disabled  SatFdbkVariant=Disabled  DerivativeFilterVariant=ForwardEulerFilter  NVariant=InternalParameters  NCopyVariant=Disabled  FilterICVariant=InternalICsFilter  IntegratorICVariant=InternalICs  ExternalResetVariant=Disabled  TRSumVariant=Passthrough  SumFdbkVariant=Disabled  SumVariant=Sum_PID  TsampFilterVariant=InternalTs  TsampNgainVariant=Passthrough  TsampIntegralVariant=Disabled_SignalSpec  ExternalSaturationOutDataTypeStr=Inherit: Same as second input  DerivativeSourceVariant=ErrorSignal  PreIntVariant=InternalPreInt
      settings: LibrarySourceBlock=simulink/Discrete/Discrete PID Controller
  Sum : Sum  Inputs=|+-
  Sum1 : Sum  Inputs=|+-
  Sum_left_error : Sum  Inputs=|+-
  Sum_right_error : Sum  Inputs=|+-
  u_left_raw : Outport
  u_right_raw : Outport  Port=2
  wires:
  Manual Switch/1 -> u_right_raw/1
  Nbar_right/1 -> Sum1/1
  PI_left/1 -> Manual Switch1/1
  Sum_left_error/1 -> PI_left/1  "left_error"
  K_left/1 -> Sum/2
  Sum_right_error/1 -> PI_right/1  "right_error"
  K_right/1 -> Sum1/2
  Nbar_left/1 -> Sum/1
  omega_right_meas/1 -> Sum_right_error/2, K_right/1
  omega_right_ref/1 -> Sum_right_error/1, Nbar_right/1
  Manual Switch1/1 -> u_left_raw/1
  PI_right/1 -> Manual Switch/2
  omega_left_meas/1 -> Sum_left_error/2, K_left/1
  Sum/1 -> Manual Switch1/2
  omega_left_ref/1 -> Nbar_left/1, Sum_left_error/1
  Sum1/1 -> Manual Switch/1

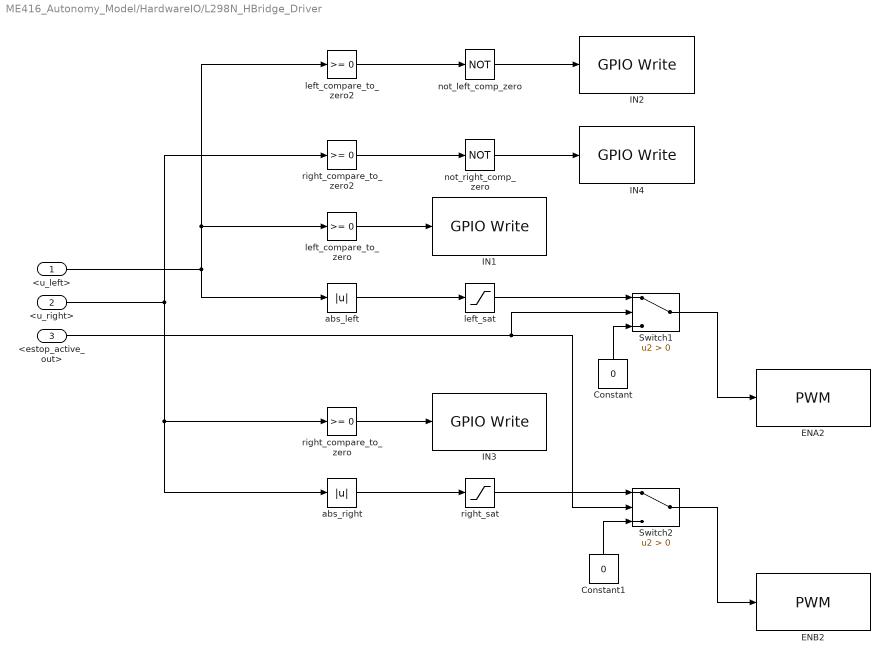
== system ME416_Autonomy_Model/HardwareIO/L298N_HBridge_Driver ==
  <u_left> : Inport
  <u_right> : Inport  Port=2
  <estop_active_out> : Inport  Port=3
  Constant : Constant  Value=0
  Constant1 : Constant  Value=0
  ENA2 : raspberrypiBasiclib/PWM  board=Pi 4 Model B  Pin_=12  Frequency=500  blockPlatform=Raspberry Pi
  ENB2 : raspberrypiBasiclib/PWM  board=Pi 4 Model B  Pin_=13  Frequency=500  blockPlatform=Raspberry Pi
  IN1 : raspberrypiBasiclib/GPIO Write  BoardProperty=Pi 4 Model B  gpio=7  blockPlatform=Raspberry Pi  PinNumber=17  board=Pi 4 Model B  direction=Output
  IN2 : raspberrypiBasiclib/GPIO Write  BoardProperty=Pi 4 Model B  gpio=5  blockPlatform=Raspberry Pi  PinNumber=17  board=Pi 4 Model B  direction=Output
  IN3 : raspberrypiBasiclib/GPIO Write  BoardProperty=Pi 4 Model B  gpio=8  blockPlatform=Raspberry Pi  PinNumber=17  board=Pi 4 Model B  direction=Output
  IN4 : raspberrypiBasiclib/GPIO Write  BoardProperty=Pi 4 Model B  gpio=6  blockPlatform=Raspberry Pi  PinNumber=17  board=Pi 4 Model B  direction=Output
  Switch1 : Switch  Criteria=u2 > Threshold  SaturateOnIntegerOverflow=off  InputSameDT=off
  Switch2 : Switch  Criteria=u2 > Threshold  SaturateOnIntegerOverflow=off  InputSameDT=off
  abs_left : Abs  SaturateOnIntegerOverflow=off
  abs_right : Abs  SaturateOnIntegerOverflow=off
  left_compare_to_zero : simulink/Logic and Bit Operations/Compare To Zero  relop=>=  OutDataTypeStr=boolean
  left_compare_to_zero2 : simulink/Logic and Bit Operations/Compare To Zero  relop=>=  OutDataTypeStr=boolean
  left_sat : Saturate  UpperLimit=1  LowerLimit=0
  not_left_comp_zero : Logic  Operator=NOT  AllPortsSameDT=off  OutDataTypeStr=boolean
  not_right_comp_zero : Logic  Operator=NOT  AllPortsSameDT=off  OutDataTypeStr=boolean
  right_compare_to_zero : simulink/Logic and Bit Operations/Compare To Zero  relop=>=  OutDataTypeStr=boolean
  right_compare_to_zero2 : simulink/Logic and Bit Operations/Compare To Zero  relop=>=  OutDataTypeStr=boolean
  right_sat : Saturate  UpperLimit=1  LowerLimit=0
  wires:
  <u_left>/1 -> left_compare_to_zero/1, left_compare_to_zero2/1, abs_left/1
  abs_right/1 -> right_sat/1
  <u_right>/1 -> right_compare_to_zero2/1, right_compare_to_zero/1, abs_right/1
  <estop_active_out>/1 -> Switch1/2, Switch2/2
  left_compare_to_zero/1 -> IN1/1
  Constant1/1 -> Switch2/3
  right_compare_to_zero2/1 -> not_right_comp_zero/1
  left_compare_to_zero2/1 -> not_left_comp_zero/1
  right_sat/1 -> Switch2/1
  not_right_comp_zero/1 -> IN4/1
  right_compare_to_zero/1 -> IN3/1
  not_left_comp_zero/1 -> IN2/1
  abs_left/1 -> left_sat/1
  Constant/1 -> Switch1/3
  left_sat/1 -> Switch1/1
  Switch1/1 -> ENA2/1
  Switch2/1 -> ENB2/1

== system ME416_Autonomy_Model/HardwareIO/LeftEncoderQuadrature ==
  Constant : Constant
  Constant1 : Constant  Value=-1
  Logical Operator : Logic  AllPortsSameDT=off  OutDataTypeStr=boolean
  Logical Operator1 : Logic  Operator=NOT  AllPortsSameDT=off  OutDataTypeStr=boolean
  Product : Product
  Sum : Sum  Inputs=|++
  Switch : Switch  Criteria=u2 > Threshold  SaturateOnIntegerOverflow=off  InputSameDT=off
  count_delay : UnitDelay  SampleTime=-1  HasFrameUpgradeWarning=on
  enc_left_phaseA : raspberrypiBasiclib/GPIO Read  BoardProperty=Pi 4 Model B  gpio=9  SampleTime=0.01  blockPlatform=Raspberry Pi  PinNumber=4  board=Pi 4 Model B  direction=Input  internalResistor=Off
  enc_left_phaseB : raspberrypiBasiclib/GPIO Read  BoardProperty=Pi 4 Model B  gpio=10  SampleTime=0.01  blockPlatform=Raspberry Pi  PinNumber=4  board=Pi 4 Model B  direction=Input  internalResistor=Off
  phaseA_delay : UnitDelay  SampleTime=-1  HasFrameUpgradeWarning=on
  enc_left_ticks : Outport
  wires:
  enc_left_phaseB/1 -> Switch/2
  Constant/1 -> Switch/1
  Logical Operator1/1 -> Logical Operator/2
  phaseA_delay/1 -> Logical Operator/1, Logical Operator1/1
  Constant1/1 -> Switch/3
  enc_left_phaseA/1 -> phaseA_delay/1
  Logical Operator/1 -> Product/1  "A_rise"
  Switch/1 -> Product/2  "dir_step"
  Product/1 -> count_delay/1, Sum/2  "delta_count"
  count_delay/1 -> Sum/1
  Sum/1 -> enc_left_ticks/1

== system ME416_Autonomy_Model/HardwareIO/RightEncoderQuadrature ==
  Constant : Constant
  Constant1 : Constant  Value=-1
  Logical Operator : Logic  AllPortsSameDT=off  OutDataTypeStr=boolean
  Logical Operator1 : Logic  Operator=NOT  AllPortsSameDT=off  OutDataTypeStr=boolean
  Product : Product
  Sum : Sum  Inputs=|++
  Switch : Switch  Criteria=u2 > Threshold  SaturateOnIntegerOverflow=off  InputSameDT=off
  count_delay : UnitDelay  SampleTime=-1  HasFrameUpgradeWarning=on
  enc_right_phaseA : raspberrypiBasiclib/GPIO Read  BoardProperty=Pi 4 Model B  gpio=11  SampleTime=0.1  blockPlatform=Raspberry Pi  PinNumber=4  board=Model B+  direction=Input  internalResistor=Off
  enc_right_phaseB : raspberrypiBasiclib/GPIO Read  BoardProperty=Pi 4 Model B  gpio=26  SampleTime=0.1  blockPlatform=Raspberry Pi  PinNumber=4  board=Model B+  direction=Input  internalResistor=Off
  phaseA_delay : UnitDelay  SampleTime=-1  HasFrameUpgradeWarning=on
  enc_right_ticks : Outport
  wires:
  Switch/1 -> Product/2  "dir_step"
  enc_right_phaseA/1 -> phaseA_delay/1
  enc_right_phaseB/1 -> Switch/2
  Constant1/1 -> Switch/3
  Constant/1 -> Switch/1
  Product/1 -> count_delay/1, Sum/2  "delta_count"
  phaseA_delay/1 -> Logical Operator/1, Logical Operator1/1
  count_delay/1 -> Sum/1
  Sum/1 -> enc_right_ticks/1
  Logical Operator1/1 -> Logical Operator/2
  Logical Operator/1 -> Product/1  "A_rise"

== system ME416_Autonomy_Model/MotionPlanner (Waypoint, Obstacle Detection)/Subsystem ==
  u_left : Inport
  u_right : Inport  Port=2
  v_meas_out : Inport  Port=3
  w_meas_out : Inport  Port=4
  estop_active_out : Inport  Port=5
  theta_hat : Inport  Port=6
  x_hat : Inport  Port=7
  y_hat : Inport  Port=8

== system ME416_Autonomy_Model/Plant/DifferentialDriveModel ==
  omega_true_left : Inport
  omega_true_right : Inport  Port=2
  Sum : Sum  Inputs=|+-
  r_L_wheel_track_Gain : Gain  Gain=r/L
  zero_pitch : Constant  Value=0
  imu_yaw_rate : Outport
  imu_pitch : Outport  Port=2
  wires:
  omega_true_right/1 -> Sum/1
  zero_pitch/1 -> imu_pitch/1
  Sum/1 -> r_L_wheel_track_Gain/1
  r_L_wheel_track_Gain/1 -> imu_yaw_rate/1
  omega_true_left/1 -> Sum/2

== system ME416_Autonomy_Model/Plant/EncoderModel ==
  omega_left_true : Inport
  omega_right_true : Inport  Port=2
  gain_counts_per_rad_left : Gain  Gain=N/(2*pi)
  gain_counts_per_rad_right : Gain  Gain=N/(2*pi)
  left_encoder_integrator : Integrator
  left_encoder_integrator1 : Integrator
  round_left_ticks : Rounding  Operator=round
  round_right_ticks : Rounding  Operator=round
  enc_left_ticks : Outport
  enc_right_ticks : Outport  Port=2
  wires:
  omega_left_true/1 -> left_encoder_integrator/1
  round_right_ticks/1 -> enc_right_ticks/1
  omega_right_true/1 -> left_encoder_integrator1/1
  left_encoder_integrator1/1 -> gain_counts_per_rad_right/1  "phi_right"
  left_encoder_integrator/1 -> gain_counts_per_rad_left/1  "phi_left"
  round_left_ticks/1 -> enc_left_ticks/1
  gain_counts_per_rad_left/1 -> round_left_ticks/1
  gain_counts_per_rad_right/1 -> round_right_ticks/1

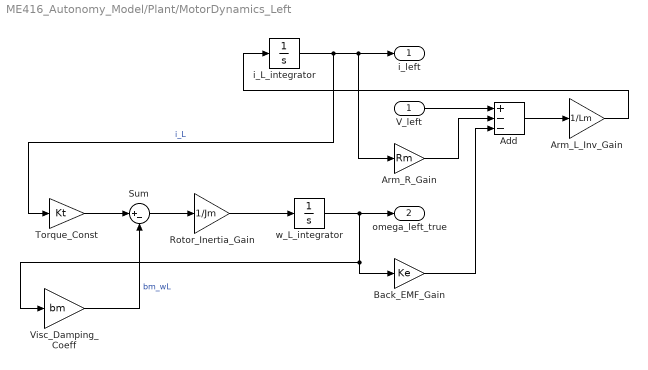
== system ME416_Autonomy_Model/Plant/MotorDynamics_Left ==
  V_left : Inport
  Add : Sum  Inputs=+--
  Arm_L_Inv_Gain : Gain  Gain=1/Lm
  Arm_R_Gain : Gain  Gain=Rm
  Back_EMF_Gain : Gain  Gain=Ke
  Rotor_Inertia_Gain : Gain  Gain=1/Jm
  Sum : Sum  Inputs=|+-
  Torque_Const : Gain  Gain=Kt
  Visc_Damping_Coeff : Gain  Gain=bm
  i_L_integrator : Integrator
  w_L_integrator : Integrator
  i_left : Outport
  "omega_left_true " : Outport  Port=2
  wires:
  V_left/1 -> Add/1
  Torque_Const/1 -> Sum/1
  Visc_Damping_Coeff/1 -> Sum/2  "bm_wL"
  w_L_integrator/1 -> Back_EMF_Gain/1, Visc_Damping_Coeff/1, "omega_left_true "/1
  Rotor_Inertia_Gain/1 -> w_L_integrator/1
  Sum/1 -> Rotor_Inertia_Gain/1
  i_L_integrator/1 -> i_left/1, Arm_R_Gain/1, Torque_Const/1  "i_L"
  Arm_R_Gain/1 -> Add/2
  Back_EMF_Gain/1 -> Add/3
  Add/1 -> Arm_L_Inv_Gain/1
  Arm_L_Inv_Gain/1 -> i_L_integrator/1

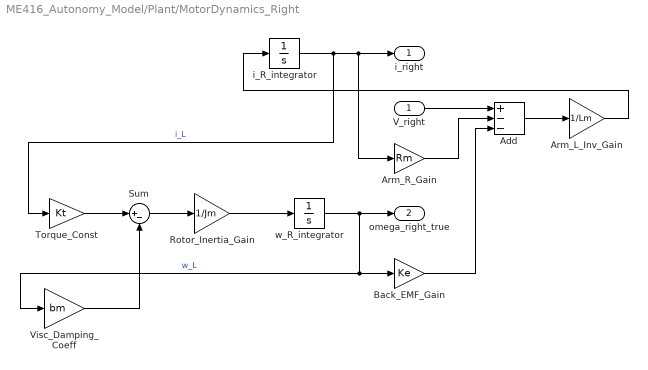
== system ME416_Autonomy_Model/Plant/MotorDynamics_Right ==
  V_right : Inport
  Add : Sum  Inputs=+--
  Arm_L_Inv_Gain : Gain  Gain=1/Lm
  Arm_R_Gain : Gain  Gain=Rm
  Back_EMF_Gain : Gain  Gain=Ke
  Rotor_Inertia_Gain : Gain  Gain=1/Jm
  Sum : Sum  Inputs=|+-
  Torque_Const : Gain  Gain=Kt
  Visc_Damping_Coeff : Gain  Gain=bm
  i_R_integrator : Integrator
  w_R_integrator : Integrator
  i_right : Outport
  "omega_right_true " : Outport  Port=2
  wires:
  V_right/1 -> Add/1
  Torque_Const/1 -> Sum/1
  Visc_Damping_Coeff/1 -> Sum/2
  w_R_integrator/1 -> Visc_Damping_Coeff/1, Back_EMF_Gain/1, "omega_right_true "/1  "w_L"
  Rotor_Inertia_Gain/1 -> w_R_integrator/1
  Sum/1 -> Rotor_Inertia_Gain/1
  i_R_integrator/1 -> i_right/1, Arm_R_Gain/1, Torque_Const/1  "i_L"
  Arm_R_Gain/1 -> Add/2
  Back_EMF_Gain/1 -> Add/3
  Add/1 -> Arm_L_Inv_Gain/1
  Arm_L_Inv_Gain/1 -> i_R_integrator/1

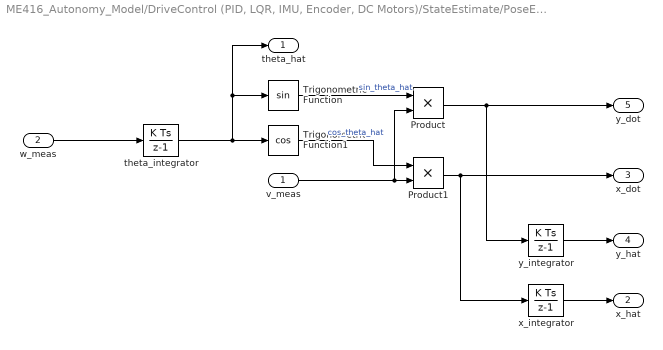
== system ME416_Autonomy_Model/DriveControl (PID, LQR, IMU, Encoder, DC Motors)/StateEstimate/PoseEstimator ==
  v_meas : Inport
  w_meas : Inport  Port=2
  Product : Product
  Product1 : Product
  Trigonometric Function : Trigonometry
  Trigonometric Function1 : Trigonometry  Operator=cos
  theta_integrator : DiscreteIntegrator  SampleTime=Ts  ICPrevOutput=DiscIntNeverNeededParam  ICPrevScaledInput=DiscIntNeverNeededParam
  x_integrator : DiscreteIntegrator  SampleTime=Ts  ICPrevOutput=DiscIntNeverNeededParam  ICPrevScaledInput=DiscIntNeverNeededParam
  y_integrator : DiscreteIntegrator  SampleTime=Ts  ICPrevOutput=DiscIntNeverNeededParam  ICPrevScaledInput=DiscIntNeverNeededParam
  theta_hat : Outport
  x_hat : Outport  Port=2
  x_dot : Outport  Port=3
  y_hat : Outport  Port=4
  y_dot : Outport  Port=5
  wires:
  Trigonometric Function/1 -> Product/1  "sin_theta_hat"
  theta_integrator/1 -> Trigonometric Function/1, theta_hat/1, Trigonometric Function1/1
  Trigonometric Function1/1 -> Product1/1  "cos_theta_hat"
  v_meas/1 -> Product/2, Product1/2
  Product/1 -> y_dot/1, y_integrator/1
  Product1/1 -> x_dot/1, x_integrator/1
  y_integrator/1 -> y_hat/1
  x_integrator/1 -> x_hat/1
  w_meas/1 -> theta_integrator/1

== matlab function ME416_Autonomy_Model/HardwareIO/MPU6050_Parse_Function ==
  data: bytes input; ax output; ay output; az output; gx output; gy output; gz output
function [ax, ay, az, gx, gy, gz] = parse_mpu6050(bytes)
%#codegen
% bytes must be a 14x1 uint8 vector read from MPU6050 starting at 0x3B
%
% Byte order:
% 1  = AX_H
% 2  = AX_L
% 3  = AY_H
% 4  = AY_L
% 5  = AZ_H
% 6  = AZ_L
% 7  = TEMP_H
% 8  = TEMP_L
% 9  = GX_H
% 10 = GX_L
% 11 = GY_H
% 12 = GY_L
% 13 = GZ_H
% 14 = GZ_L

% Convert byte pairs to unsigned 16-bit
ax_u = bitor(bitshift(uint16(bytes(1)), 8), uint16(bytes(2)));
ay_u = bitor(bitshift(uint16(bytes(3)), 8), uint16(bytes(4)));
az_u = bitor(bitshift(uint16(bytes(5)), 8), uint16(bytes(6)));

gx_u = bitor(bitshift(uint16(bytes(9)), 8), uint16(bytes(10)));
gy_u = bitor(bitshift(uint16(bytes(11)), 8), uint16(bytes(12)));
gz_u = bitor(bitshift(uint16(bytes(13)), 8), uint16(bytes(14)));

% Convert unsigned to signed
ax_raw = toSigned16(ax_u);
ay_raw = toSigned16(ay_u);
az_raw = toSigned16(az_u);

gx_raw = toSigned16(gx_u);
gy_raw = toSigned16(gy_u);
gz_raw = toSigned16(gz_u);

% Scale to physical units
% Assumes accel +/-2g and gyro +/-250 deg/s
ax = ax_raw / 16384.0;
ay = ay_raw / 16384.0;
az = az_raw / 16384.0;

gx = (gx_raw / 131.0) * (pi / 180.0);
gy = (gy_raw / 131.0) * (pi / 180.0);
gz = (gz_raw / 131.0) * (pi / 180.0);

end

function x = toSigned16(u)
% Convert uint16 to signed value stored as double
if u >= 32768
    x = double(int32(u) - 65536);
else
    x = double(u);
end
end

== matlab function ME416_Autonomy_Model/HardwareIO/IMU1_Kalman_Filter ==
  data: ax_parsed input; ax_kf output; ay_parsed input; az_parsed input; gx_parsed input; ay_kf output; az_kf output; pitch_kf output; roll_kf output; yaw_rate_kf output; gy_parsed input; gz_parsed input
function [ax_kf, ay_kf, az_kf, pitch_kf, roll_kf, yaw_rate_kf] = imu_kalman_filter(ax_parsed, ay_parsed, az_parsed, gx_parsed, gy_parsed, gz_parsed)
%#codegen
% Simple 1D Kalman smoothing filter for IMU signals
%
% Inputs:
%   ax, ay, az   -> accelerometer in g
%   gx, gy, gz   -> gyro in rad/sa
%
% Outputs:
%   ax_f, ay_f, az_f     -> filtered accel
%   pitch_f, roll_f      -> filtered angles from accel
%   yaw_rate_f           -> filtered yaw rate from gyro z

% Persistent states for each filtered signal
persistent x_ax_parsed p_ax_parsed
persistent x_ay_parsed p_ay_parsed
persistent x_az_parsed p_az_parsed
persistent x_pitch p_pitch
persistent x_roll p_roll
persistent x_yaw p_yaw

% Tunable Kalman parameters
% Lower q = smoother/slower
% Lower r = trusts measurement more
q_acc = 0.01;
r_acc = 0.1;

q_ang = 0.01;
r_ang = 0.1;

q_yaw = 0.05;
r_yaw = 0.2;

% Compute raw roll/pitch from accelerometer
roll_meas  = atan2(ay_parsed, az_parsed);
pitch_meas = atan2(-ax_parsed, sqrt(ay_parsed^2 + az_parsed^2));

% Initialize on first run
if isempty(x_ax_parsed)
    x_ax_parsed = ax_parsed;      p_ax_parsed = 1.0;
    x_ay_parsed = ay_parsed;      p_ay_parsed = 1.0;
    x_az_parsed = az_parsed;      p_az_parsed = 1.0;

    x_roll  = roll_meas;    p_roll  = 1.0;
    x_pitch = pitch_meas;   p_pitch = 1.0;

    x_yaw = gz_parsed;      p_yaw = 1.0;
end

% Filter accel channels
[x_ax_parsed, p_ax_parsed] = kalman_update(x_ax_parsed, p_ax_parsed, ax_parsed, q_acc, r_acc);
[x_ay_parsed, p_ay_parsed] = kalman_update(x_ay_parsed, p_ay_parsed, ay_parsed, q_acc, r_acc);
[x_az_parsed, p_az_parsed] = kalman_update(x_az_parsed, p_az_parsed, az_parsed, q_acc, r_acc);

% Filter roll/pitch angles
[x_roll, p_roll]   = kalman_update(x_roll, p_roll, roll_meas, q_ang, r_ang);
[x_pitch, p_pitch] = kalman_update(x_pitch, p_pitch, pitch_meas, q_ang, r_ang);

% Filter yaw rate (gyro z)
[x_yaw, p_yaw] = kalman_update(x_yaw, p_yaw, gz_parsed, q_yaw, r_yaw);

% Outputs
ax_kf = x_ax_parsed;
ay_kf = x_ay_parsed;
az_kf = x_az_parsed;

roll_kf     = x_roll;
pitch_kf    = x_pitch;
yaw_rate_kf = x_yaw;

end

function [x, p] = kalman_update(x, p, z, q, r)
% 1D Kalman filter update

% Prediction
p = p + q;

% Correction
k = p / (p + r);
x = x + k * (z - x);
p = (1 - k) * p;

end
